simulink model "model"  (R2021b)
settings: Solver=VariableStepAuto  StartTime=0.0  StopTime=10.0  RelTol=1e-3
libraries: simulink x1
settings Model: Creator=O  LastModifiedBy=user2

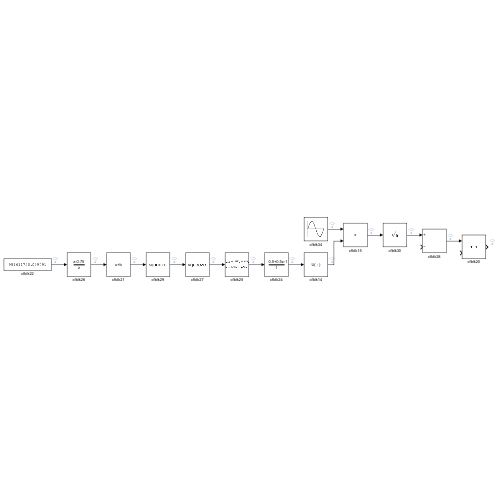
[thumbnail: Simulink's stored preview of the top-level diagram]
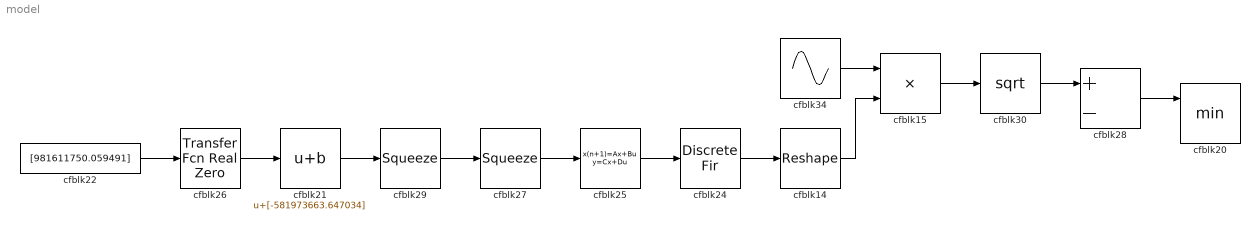
== system model ==
  cfblk14 : Reshape
  cfblk15 : Product  Inputs=**  OutDataTypeStr=double
  cfblk20 : MinMax  Inputs=2  OutDataTypeStr=double
  cfblk21 : Bias  Bias=[-581973663.647034]
  cfblk22 : Constant  Value=[981611750.059491]  OutDataTypeStr=double  SampleTime=1
  cfblk24 : DiscreteFir  SampleTime=1
  cfblk25 : DiscreteStateSpace
  cfblk26 : simulink/Discrete/Transfer Fcn Real Zero  ZeroZ=0.75  ICPrevInput=0.0  DoSatur=off
      settings: SourceProductBaseCode=SL
  cfblk27 : Squeeze
  cfblk28 : Sum  Inputs=+-  OutDataTypeStr=double
  cfblk29 : Squeeze
  cfblk30 : Sqrt  OutDataTypeStr=double  SaturateOnIntegerOverflow=on
  cfblk34 : Sin  Amplitude=[668262176.314761]  Bias=[-551335817.625013]  SampleTime=0
  wires:
  cfblk27/1 -> cfblk25/1
  cfblk25/1 -> cfblk24/1
  cfblk15/1 -> cfblk30/1
  cfblk14/1 -> cfblk15/2
  cfblk28/1 -> cfblk20/1
  cfblk26/1 -> cfblk21/1
  cfblk24/1 -> cfblk14/1
  cfblk34/1 -> cfblk15/1
  cfblk30/1 -> cfblk28/1
  cfblk29/1 -> cfblk27/1
  cfblk21/1 -> cfblk29/1
  cfblk22/1 -> cfblk26/1
